simulink model "final"  (R2024a)
settings: Solver=FixedStepAuto  StartTime=0.0  StopTime=80  FixedStep=1e-3  RelTol=1e-3
undefined symbols (not defined in the file): k1, k2, k3, k4, k5
libraries: simulink x1
settings Model: Creator=dario  LastModifiedBy=juanj
settings RTWCC: GPUComputeCapability=3.5

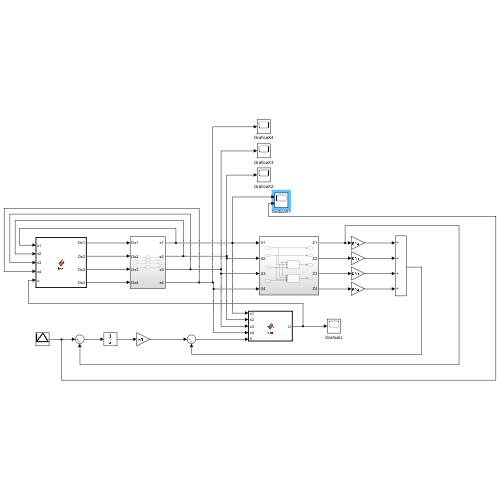
[thumbnail: Simulink's stored preview of the top-level diagram]
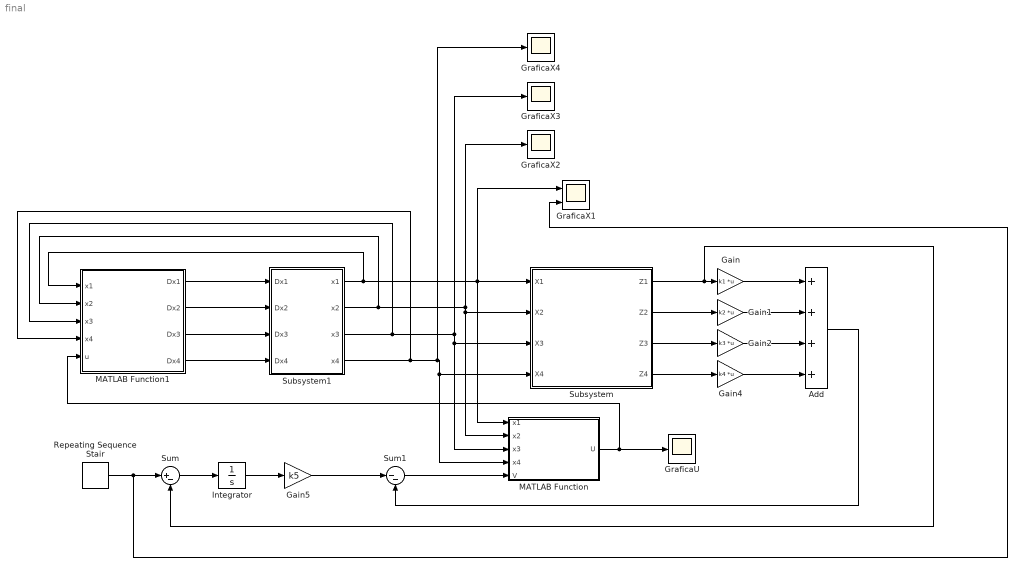
== system final ==
  Add : Sum  Inputs=++++
  Gain : Gain  Gain=k1  Multiplication=Matrix(K*u)
  Gain1 : Gain  Gain=k2  Multiplication=Matrix(K*u)
  Gain2 : Gain  Gain=k3  Multiplication=Matrix(K*u)
  Gain4 : Gain  Gain=k4  Multiplication=Matrix(K*u)
  Gain5 : Gain  Gain=k5
  GraficaU : Scope
  GraficaX1 : Scope  NumInputPorts=2
  GraficaX2 : Scope
  GraficaX3 : Scope
  GraficaX4 : Scope
  Integrator : Integrator
  MATLAB Function : MATLAB Function  TreatAsAtomicUnit=on
  MATLAB Function1 : MATLAB Function  TreatAsAtomicUnit=on
  Repeating Sequence Stair : simulink/Sources/Repeating Sequence Stair  OutValues=inter'  tsamp=4  OutMin=[]  OutMax=[]  OutDataTypeStr=double  OutputDataTypeScalingMode=double  OutDataType=fixdt(0,8)  ConRadixGroup=Best Precision: Vector-wise  OutScaling=2^-12
  Subsystem : Subsystem
  Subsystem1 : Subsystem
  Sum : Sum  Inputs=|+-
  Sum1 : Sum  Inputs=|--
  wires:
  Subsystem1/1(x1) -> GraficaX1/1, MATLAB Function/1(x1), Subsystem/1(X1), MATLAB Function1/1(x1)
  Subsystem1/2(x2) -> Subsystem/2(X2), MATLAB Function/2(x2), GraficaX2/1, MATLAB Function1/2(x2)
  Subsystem1/3(x3) -> MATLAB Function/3(x3), Subsystem/3(X3), GraficaX3/1, MATLAB Function1/3(x3)
  Subsystem1/4(x4) -> GraficaX4/1, MATLAB Function/4(x4), Subsystem/4(X4), MATLAB Function1/4(x4)
  Subsystem/1(Z1) -> Sum/2, Gain/1
  Subsystem/2(Z2) -> Gain1/1
  Subsystem/3(Z3) -> Gain2/1
  Subsystem/4(Z4) -> Gain4/1
  Gain/1 -> Add/1
  Gain4/1 -> Add/4
  Gain2/1 -> Add/3
  Gain1/1 -> Add/2
  Sum/1 -> Integrator/1
  Integrator/1 -> Gain5/1
  Gain5/1 -> Sum1/1
  Add/1 -> Sum1/2
  Sum1/1 -> MATLAB Function/5(V)
  MATLAB Function1/1(Dx1) -> Subsystem1/1(Dx1)
  MATLAB Function1/2(Dx2) -> Subsystem1/2(Dx2)
  MATLAB Function1/3(Dx3) -> Subsystem1/3(Dx3)
  MATLAB Function1/4(Dx4) -> Subsystem1/4(Dx4)
  MATLAB Function/1(U) -> GraficaU/1, MATLAB Function1/5(u)
  Repeating Sequence Stair/1 -> GraficaX1/2, Sum/1

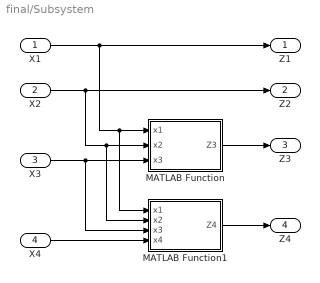
== system final/Subsystem ==
  X1 : Inport
  X2 : Inport  Port=2
  X3 : Inport  Port=3
  X4 : Inport  Port=4
  MATLAB Function : MATLAB Function  TreatAsAtomicUnit=on
  MATLAB Function1 : MATLAB Function  TreatAsAtomicUnit=on
  Z1 : Outport
  Z2 : Outport  Port=2
  Z3 : Outport  Port=3
  Z4 : Outport  Port=4
  wires:
  X1/1 -> MATLAB Function1/1(x1), MATLAB Function/1(x1), Z1/1
  MATLAB Function/1(Z3) -> Z3/1
  X2/1 -> MATLAB Function1/2(x2), MATLAB Function/2(x2), Z2/1
  X3/1 -> MATLAB Function1/3(x3), MATLAB Function/3(x3)
  MATLAB Function1/1(Z4) -> Z4/1
  X4/1 -> MATLAB Function1/4(x4)

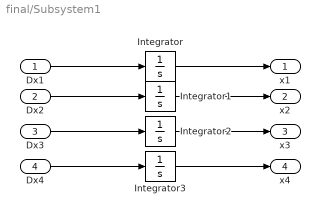
== system final/Subsystem1 ==
  Dx1 : Inport
  Dx2 : Inport  Port=2
  Dx3 : Inport  Port=3
  Dx4 : Inport  Port=4
  Integrator{,1..3} (4 alike) : Integrator
  x1 : Outport
  x2 : Outport  Port=2
  x3 : Outport  Port=3
  x4 : Outport  Port=4
  wires:
  Dx1/1 -> Integrator/1
  Integrator/1 -> x1/1
  Integrator1/1 -> x2/1
  Dx2/1 -> Integrator1/1
  Integrator2/1 -> x3/1
  Dx3/1 -> Integrator2/1
  Integrator3/1 -> x4/1
  Dx4/1 -> Integrator3/1

== matlab function final/Subsystem/MATLAB Function1 ==
  data: x1 input; Z4 output; x2 input; x3 input; x4 input
function Z4 = fcn(x1,x2,x3,x4)
T1=0.3; 
Mg=0.0383; 
a1=0.105; 
b1=9.36e-3; 
I=4.37e-3;
B=1.84e-3;

Z4 = (B*(- a1*x3^2 - b1*x3 + B*x2 + Mg*sin(x1)))/I^(2) - ((x3 - x4)*(b1 + 2*a1*x3))/(I*T1) - (Mg*x2*cos(x1))/I;

== matlab function final/Subsystem/MATLAB Function ==
  data: x1 input; Z3 output; x2 input; x3 input
function Z3 = fcn(x1,x2,x3)
 
Mg=0.0383; 
a1=0.105; 
b1=9.36e-3; 
I=4.37e-3;
B=1.84e-3;

Z3 = -(- a1*x3^2 - b1*x3 + B*x2 + Mg*sin(x1))/I ;

== matlab function final/MATLAB Function ==
  data: x1 input; U output; x2 input; x3 input; x4 input; V input
function U = fcn(x1,x2,x3,x4,V)
T1=0.3; 
Mg=0.0383; 
a1=0.105; 
b1=9.36e-3; 
I=4.37e-3;
B=1.84e-3;
U = (I*T1^2*(V + ((B^2 - I*Mg*cos(x1))*(- a1*x3^2 - b1*x3 + B*x2 + Mg*sin(x1)))/I^(3) + (x4*(b1 + 2*a1*x3))/(I*T1^2) - (Mg*x2*(B*cos(x1) + I*x2*sin(x1)))/I^(2) - ((x3 - x4)*(I*b1 + B*T1*b1 + 4*I*a1*x3 - 2*I*a1*x4 + 2*B*T1*a1*x3))/(I^(2)*T1^2)))/(b1 + 2*a1*x3);

== matlab function final/MATLAB Function1 ==
  data: x1 input; Dx1 output; x2 input; x3 input; x4 input; Dx2 output; u input; Dx3 output; Dx4 output
function [Dx1,Dx2,Dx3,Dx4]= fcn(x1,x2,x3,x4,u)

T1=0.3; 
Mg=0.0383; 
a1=0.105; 
b1=9.36e-3; 
I=4.37e-3;
B=1.84e-3;

Dx1=x2;
Dx2=-(- a1*x3^2 - b1*x3 + B*x2 + Mg*sin(x1))/I;
Dx3=-(x3 - x4)/T1 ;
Dx4=(u - x4)/T1;
